simulink model "Lab1_adaptive_v0"  (R2022b)
settings: Solver=VariableStepAuto  StartTime=0.0  StopTime=t  MaxStep=0.01  RelTol=1e-3
undefined symbols (not defined in the file): gamma, lambda, theta
settings Model: Creator=DuPont  LastModifiedBy=DuPont

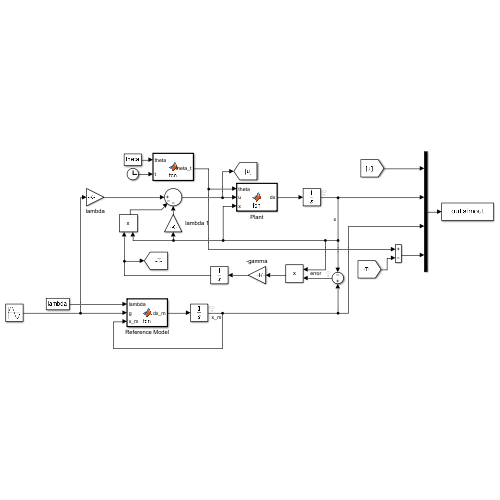
[thumbnail: Simulink's stored preview of the top-level diagram]
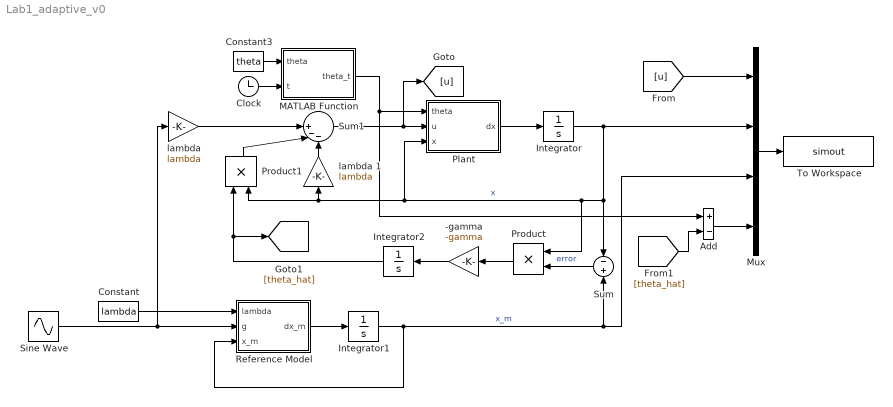
== system Lab1_adaptive_v0 ==
  -gamma : Gain  Gain=-gamma
  Add : Sum  Inputs=+-
  Clock : Clock
  Constant : Constant  Value=lambda
  Constant3 : Constant  Value=theta
  Integrator : Integrator
  Integrator1 : Integrator
  Integrator2 : Integrator
  MATLAB Function : MATLAB Function  TreatAsAtomicUnit=on
  Mux : Mux
  Plant : MATLAB Function  TreatAsAtomicUnit=on
  Product : Product
  Product1 : Product
  Reference Model : MATLAB Function  TreatAsAtomicUnit=on
  Sine Wave : Sin  Bias=2  Frequency=8  SampleTime=0
  Sum : Sum  Inputs=-|+
  Sum1 : Sum  Inputs=||+--
  To Workspace : ToWorkspace  VariableName=simout  SaveFormat=Structure With Time  SampleTime=-1
  lambda : Gain  Gain=lambda
  lambda 1 : Gain  Gain=lambda
  wires:
  Plant/1(dx) -> Integrator/1
  Integrator/1 -> Sum/1, Product/1, Product1/2, lambda 1/1, Plant/3(x), Mux/2  "x"
  Reference Model/1(dx_m) -> Integrator1/1
  Integrator1/1 -> Mux/3, Sum/2, Reference Model/3(x_m)  "x_m"
  Sum/1 -> Product/2  "error"
  Product/1 -> -gamma/1
  -gamma/1 -> Integrator2/1
  Integrator2/1 -> [theta_hat], Product1/1
  Constant/1 -> Reference Model/1(lambda)
  Sine Wave/1 -> lambda/1, Reference Model/2(g)
  Sum1/1 -> [u], Plant/2(u)
  Product1/1 -> Sum1/2
  lambda/1 -> Sum1/1
  lambda 1/1 -> Sum1/3
  [u] -> Mux/1
  Add/1 -> Mux/4
  MATLAB Function/1(theta_t) -> Plant/1(theta), Add/1
  [theta_hat] -> Add/2
  Mux/1 -> To Workspace/1
  Clock/1 -> MATLAB Function/2(t)
  Constant3/1 -> MATLAB Function/1(theta)

== matlab function Lab1_adaptive_v0/Plant ==
  data: theta input; u input; x input; dx output
function dx = fcn(theta, u, x)

dx = theta*x + u;

== matlab function Lab1_adaptive_v0/MATLAB Function ==
  data: theta input; theta_t output; t input
function theta_t = fcn(theta, t)

if t < 10
    theta_t = theta;
else 
    theta_t = theta*3;
end

== matlab function Lab1_adaptive_v0/Reference Model ==
  data: lambda input; dx_m output; g input; x_m input
function dx_m = fcn(lambda, g, x_m)

dx_m = -lambda*x_m + lambda*g;
